simulink model "erc_mission_node"  (R2026a)
settings: Solver=FixedStepDiscrete  FixedStep=1/15  EnableMultiTasking=on
libraries: ros2lib x4
settings Model: Creator=Marko  LastModifiedBy=Marko
settings SolverCC: PositivePriorityOrder=on
settings OptimizationCC: InitFltsAndDblsToZero=on
settings HardwareCC: ProdBitPerLong=64.0  ProdLargestAtomicInteger=LongLong  ProdLargestAtomicFloat=Double  ProdHWDeviceType=ARM Compatible->ARM Cortex-A (64-bit)  TargetLongLongMode=on
settings RTWCC: SystemTargetFile=ert.tlc  HardwareBoard=Robot Operating System 2 (ROS 2)  TLCOptions="-aInlineSetEventsForThisBaseRateFcn=TLC_FALSE -aSuppressMultiTaskScheduler=TLC_FALSE  -aRateBasedStepFcn=0"  Toolchain=Colcon Tools  BuildConfiguration=Faster Runs  TargetLang=C++  Description=Embedded Coder
settings ERTTargetCC: ExtModeTransport=2.0  ExtModeAutomaticAllocSize=off  RootIOFormat=Structure reference  CodeInterfacePackaging=C++ class  SubcomponentCodeInterfacePackaging=C++ class

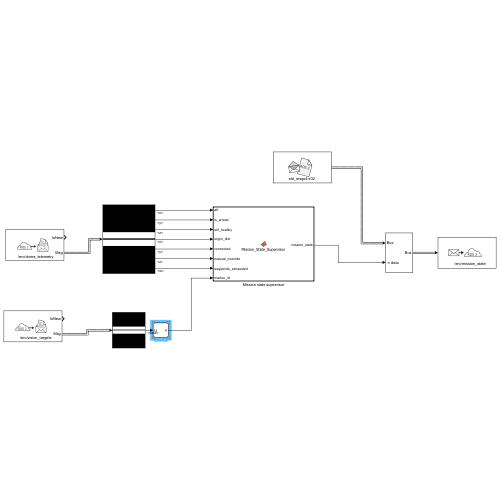
[thumbnail: Simulink's stored preview of the top-level diagram]
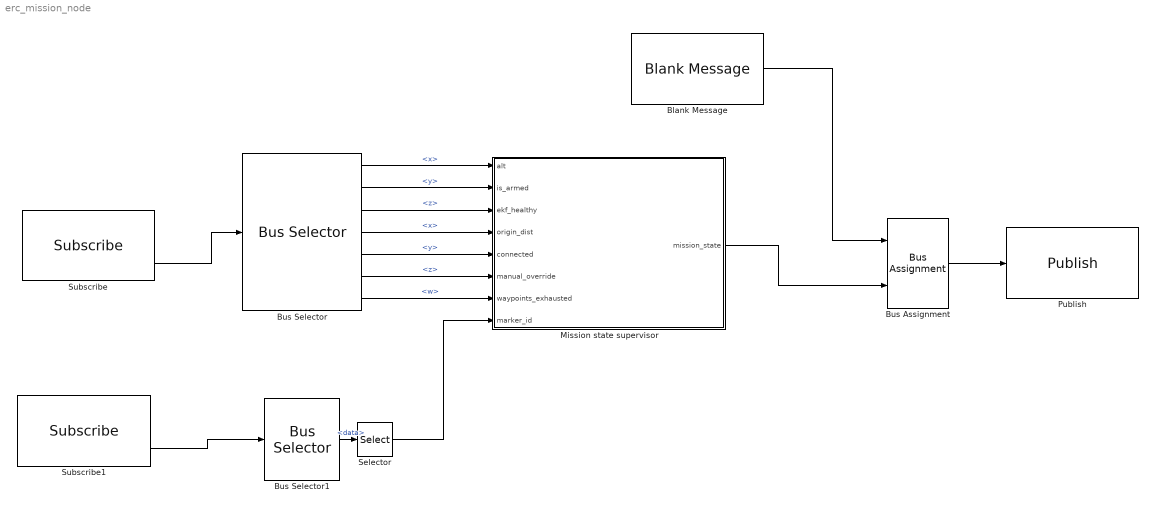
== system erc_mission_node ==
  Blank Message : ros2lib/Blank Message  messageClass=Message  entityType=std_msgs/Int32  messageType=std_msgs/Int32  SampleTime=inf
  Bus Assignment : BusAssignment  AssignedSignals=data
  Bus Selector : BusSelector  OutputSignals=position.x,position.y,position.z,orientation.x,orientation.y,orientation.z,orientation.w
  Bus Selector1 : BusSelector  OutputSignals=data
  Mission state supervisor : MATLAB Function  TreatAsAtomicUnit=on
  Publish : ros2lib/Publish  topicSource=Specify your own  topic=/erc/mission_state  messageType=std_msgs/Int32  QOSHistory=Keep last  QOSDepth=10  QOSReliability=Reliable  QOSDurability=Volatile  QOSDeadline=Inf  QOSLifespan=Inf  QOSLiveliness=Automatic  QOSLeaseDuration=Inf  QOSAvoidROSNamespaceConventions=off
  Selector : Selector  IndexOptions=Index vector (dialog)  Indices=1  OutputSizes=1
  Subscribe : ros2lib/Subscribe  topicSource=Specify your own  topic=/erc/drone_telemetry  messageType=geometry_msgs/Pose  sampleTime=-1  QOSHistory=Keep last  QOSDepth=10  QOSReliability=Reliable  QOSDurability=Volatile  QOSDeadline=Inf  QOSLifespan=Inf  QOSLiveliness=Automatic  QOSLeaseDuration=Inf  QOSAvoidROSNamespaceConventions=off
  Subscribe1 : ros2lib/Subscribe  topicSource=Specify your own  topic=/erc/vision_targets  messageType=std_msgs/Float64MultiArray  sampleTime=-1  QOSHistory=Keep last  QOSDepth=10  QOSReliability=Reliable  QOSDurability=Volatile  QOSDeadline=Inf  QOSLifespan=Inf  QOSLiveliness=Automatic  QOSLeaseDuration=Inf  QOSAvoidROSNamespaceConventions=off
  wires:
  Subscribe/2 -> Bus Selector/1
  Bus Selector/1 -> Mission state supervisor/1(alt)  "<x>"
  Bus Selector/2 -> Mission state supervisor/2(is_armed)  "<y>"
  Bus Selector/3 -> Mission state supervisor/3(ekf_healthy)  "<z>"
  Bus Selector/4 -> Mission state supervisor/4(origin_dist)  "<x>"
  Bus Selector/5 -> Mission state supervisor/5(connected)  "<y>"
  Bus Selector/6 -> Mission state supervisor/6(manual_override)  "<z>"
  Bus Selector/7 -> Mission state supervisor/7(waypoints_exhausted)  "<w>"
  Subscribe1/2 -> Bus Selector1/1
  Bus Selector1/1 -> Selector/1  "<data>"
  Blank Message/1 -> Bus Assignment/1
  Mission state supervisor/1(mission_state) -> Bus Assignment/2
  Bus Assignment/1 -> Publish/1
  Selector/1 -> Mission state supervisor/8(marker_id)

== matlab function erc_mission_node/Mission state supervisor ==
  data: alt input; mission_state output; is_armed input; ekf_healthy input; origin_dist input; connected input; manual_override input; waypoints_exhausted input; marker_id input
function mission_state = Mission_State_Supervisor(alt, is_armed, ekf_healthy, origin_dist, connected, manual_override, waypoints_exhausted, marker_id)
%#codegen
% =========================================================================
% ERC 2026 DRONING SUB-TASK: FULL HIGH-LEVEL SUPERVISORY STATE MACHINE
%
% States (int32):
%   0 = IDLE       (Preflight checks & EKF convergence)
%   1 = TAKEOFF    (Arming & climb to 1.5m)
%   2 = SEARCH     (Marker scanning sweep)
%   3 = DESCEND    (Precision landing approach & touchdown)
%   4 = COMPLETE   (Touchdown confirmed, disarmed, or pilot override)
% =========================================================================

    % ---------------------------------------------------------------------
    % Persistent State Variables (Preserved across time steps)
    % ---------------------------------------------------------------------
    persistent current_state;
    persistent state_timer_s;
    persistent detect_confirm_ticks;
    persistent marker_last_seen_timer_s;

    % Sampling period: dt = 1/15s (matching 15 Hz model rate)
    dt = 1.0 / 15.0;

    % ---------------------------------------------------------------------
    % Tunable Parameters & Thresholds
    % ---------------------------------------------------------------------
    TARGET_ALT_M            = 1.5;     % Takeoff target altitude
    TAKEOFF_ALT_COEFF       = 0.85;    % 85% of target (1.275 m)
    TOUCHDOWN_ALT_M         = 0.25;    % Ground detection threshold
    REQUIRED_CONFIRM_TICKS  = int32(15); % Consecutive detection frames (~330ms)

    MAX_ORIGIN_DRIFT_IDLE_M = 6.0;     % Max drift allowed while on pad before takeoff
    GEOFENCE_MAX_DIST_M     = 8.0;     % Max distance from origin before emergency LAND

    TIMEOUT_TAKEOFF_S       = 30.0;    % Max takeoff climb duration
    TIMEOUT_SEARCH_S        = 320.0;   % Max search duration
    TIMEOUT_DESCEND_S       = 30.0;    % Max descent duration

    % ---------------------------------------------------------------------
    % Initialization (First execution step)
    % ---------------------------------------------------------------------
    if isempty(current_state)
        current_state            = int32(0); % Start in IDLE
        state_timer_s            = 0.0;
        detect_confirm_ticks     = int32(0);
        marker_last_seen_timer_s = 0.0;
    end

    % Advance state timer
    state_timer_s = state_timer_s + dt;

    % ---------------------------------------------------------------------
    % 1. Global Safety Checks (Override & Geofence)
    % ---------------------------------------------------------------------
    % Pilot Manual Override: Instantly switch to COMPLETE and yield control
    if manual_override > 0.5 && current_state ~= int32(4)
        current_state = int32(4); % COMPLETE (Autonomy disengaged)
        state_timer_s = 0.0;
    end

    % Geofence Breach: If drone drifts outside arena (> 8m), force landing
    if origin_dist > GEOFENCE_MAX_DIST_M && current_state ~= int32(0) && current_state ~= int32(4)
        current_state = int32(3); % DESCEND (LAND)
        state_timer_s = 0.0;
    end

    % ---------------------------------------------------------------------
    % 2. Marker Detection Tracking & Debounce
    % ---------------------------------------------------------------------
    if marker_id == 102
        detect_confirm_ticks     = detect_confirm_ticks + int32(1);
        marker_last_seen_timer_s = 0.0;
    else
        detect_confirm_ticks     = max(detect_confirm_ticks-2, 0);
        marker_last_seen_timer_s = marker_last_seen_timer_s + dt;
    end

    % ---------------------------------------------------------------------
    % 3. State Machine Transitions
    % ---------------------------------------------------------------------
    switch current_state

        case 0 % ==================== IDLE ====================
            % Guard: Pixhawk connected, EKF healthy, and origin stable on pad
            if (connected > 0.5) && (ekf_healthy > 0.5) && (origin_dist <= MAX_ORIGIN_DRIFT_IDLE_M)
                current_state = int32(1); % Transition -> TAKEOFF
                state_timer_s = 0.0;
            end

        case 1 % ==================== TAKEOFF ====================
            % Guard 1: Altitude reached 85% of target (1.275m)
            if alt >= (TARGET_ALT_M * TAKEOFF_ALT_COEFF)
                current_state = int32(2); % Transition -> SEARCH
                state_timer_s = 0.0;
            % Guard 2: Takeoff timeout failsafe (30s) -> Abort to landing
            elseif state_timer_s > TIMEOUT_TAKEOFF_S
                current_state = int32(3); % Transition -> DESCEND (LAND)
                state_timer_s = 0.0;
            end

        case 2 % ==================== SEARCH ====================
            % Guard 1: Marker 102 confirmed (5 consecutive frames)
            if detect_confirm_ticks >= REQUIRED_CONFIRM_TICKS
                current_state = int32(3); % Transition -> DESCEND (Precision Land)
                state_timer_s = 0.0;
            % Guard 2: Search timeout failsafe (320s) OR waypoints exhausted -> Abort to landing
            elseif (state_timer_s > TIMEOUT_SEARCH_S) || (waypoints_exhausted > 0.5)
                current_state = int32(3); % Transition -> DESCEND (LAND)
                state_timer_s = 0.0;
            end

        case 3 % ==================== DESCEND ====================
            % Guard 1: Normal Touchdown (alt < 0.25m AND motors disarmed)
            if (alt < TOUCHDOWN_ALT_M) && (is_armed < 0.5)
                current_state = int32(4); % Transition -> COMPLETE
                state_timer_s = 0.0;

            % Guard 2: Marker-Lost Abort (lost > 3s while above 1.0m) -> Climb back to SEARCH
            %elseif (marker_last_seen_timer_s > 3.0) && (alt > 1.0) && (state_timer_s > 2.0)
            %    current_state = int32(2); % Transition -> SEARCH
            %    state_timer_s = 0.0;

            % Guard 3: Descent timeout (30s) -> Force completion once disarmed
            elseif (state_timer_s > TIMEOUT_DESCEND_S) && (is_armed < 0.5)
                current_state = int32(4); % Transition -> COMPLETE
                state_timer_s = 0.0;
            end

        case 4 % ==================== COMPLETE ====================
            % Mission successfully finished or disengaged
            current_state = int32(4);

        otherwise
            current_state = int32(0);
    end

    % Output the active mission state
    mission_state = current_state;
end
